simulink model "ex3_2"  (R2015b)
settings: Solver=VariableStepAuto  StartTime=0.0  StopTime=50.0  RelTol=1e-3
settings Model: Creator=ovi  LastModifiedBy=ovi

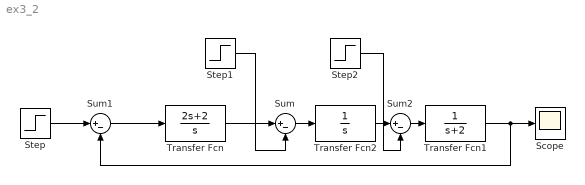
== system ex3_2 ==
  Scope : Scope
  Step : Step  SampleTime=0
  Step1 : Step  Time=3  After=0.2  SampleTime=0
  Step2 : Step  Time=6  After=0.2  SampleTime=0
  Sum : Sum  Inputs=|+-
  Sum1 : Sum  Inputs=|+-
  Sum2 : Sum  Inputs=|+-
  Transfer Fcn : TransferFcn  Numerator=[2 2]  Denominator=[1 0]
  Transfer Fcn1 : TransferFcn  Denominator=[1 2]
  Transfer Fcn2 : TransferFcn  Denominator=[1 0]
  wires:
  Transfer Fcn/1 -> Sum/1
  Sum/1 -> Transfer Fcn2/1
  Transfer Fcn2/1 -> Sum2/1
  Sum2/1 -> Transfer Fcn1/1
  Step1/1 -> Sum/2
  Step2/1 -> Sum2/2
  Step/1 -> Sum1/1
  Transfer Fcn1/1 -> Sum1/2, Scope/1
  Sum1/1 -> Transfer Fcn/1
